simulink library "linearPlnt_cl"  (R2018a)
settings: Solver=VariableStepAuto  StartTime=0.0  StopTime=10.0  RelTol=1e-3
libraries: linearPlnt_ul x1
settings Model: Creator=mcobb  LastModifiedBy=mcobb

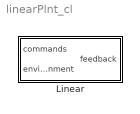
== system linearPlnt_cl ==
  Linear : Subsystem

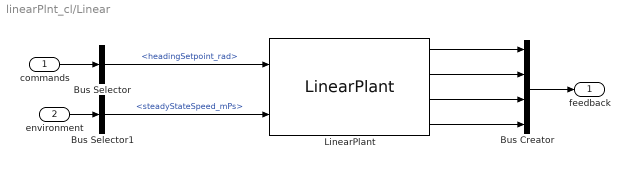
== system linearPlnt_cl/Linear ==
  commands : Inport
  environment : Inport  Port=2
  Bus Creator : BusCreator  Inputs=4
  Bus Selector : BusSelector  OutputSignals=headingSetpoint_rad
  Bus Selector1 : BusSelector  OutputSignals=steadyStateSpeed_mPs
  LinearPlant : linearPlnt_ul/LinearPlant
  feedback : Outport
  wires:
  Bus Selector/1 -> LinearPlant/1  "<headingSetpoint_rad>"
  Bus Selector1/1 -> LinearPlant/2  "<steadyStateSpeed_mPs>"
  commands/1 -> Bus Selector/1
  environment/1 -> Bus Selector1/1
  LinearPlant/4 -> Bus Creator/4
  LinearPlant/3 -> Bus Creator/3
  Bus Creator/1 -> feedback/1
  LinearPlant/2 -> Bus Creator/2
  LinearPlant/1 -> Bus Creator/1
